simulink model "model"  (R2022a)
settings: Solver=VariableStepAuto  StartTime=0.0  StopTime=Inf  RelTol=1e-3
settings Model: Creator=mateu  LastModifiedBy=mateu

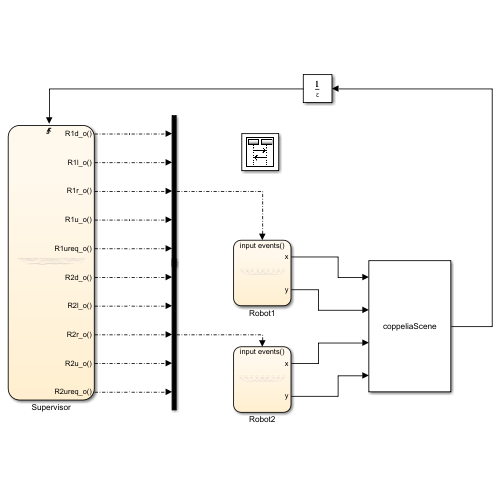
[thumbnail: Simulink's stored preview of the top-level diagram]
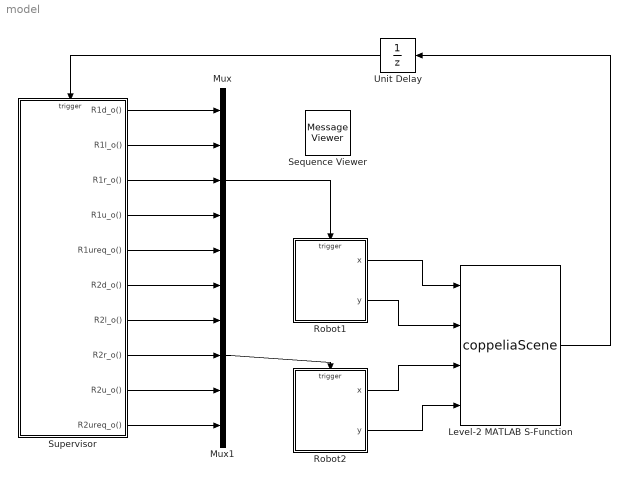
== system model ==
  Level-2 MATLAB S-Function : M-S-Function  FunctionName=coppeliaScene
  Mux : Mux  Inputs=5
  Mux1 : Mux  Inputs=5
  Robot1 : Stateflow chart  TreatAsAtomicUnit=on
  Robot2 : Stateflow chart  TreatAsAtomicUnit=on
  Sequence Viewer : MessageViewer
  Supervisor : Stateflow chart  TreatAsAtomicUnit=on
  Unit Delay : UnitDelay  SampleTime=-1  HasFrameUpgradeWarning=on
  wires:
  Level-2 MATLAB S-Function/1 -> Unit Delay/1
  Robot2/1(x) -> Level-2 MATLAB S-Function/3
  Robot2/2(y) -> Level-2 MATLAB S-Function/4
  Robot1/1(x) -> Level-2 MATLAB S-Function/1
  Robot1/2(y) -> Level-2 MATLAB S-Function/2
  Unit Delay/1 -> Supervisor/Trigger
  Mux/1 -> Robot1/Trigger
  Mux1/1 -> Robot2/Trigger
  Supervisor/1(R1d_o()) -> Mux/1
  Supervisor/2(R1l_o()) -> Mux/2
  Supervisor/3(R1r_o()) -> Mux/3
  Supervisor/4(R1u_o()) -> Mux/4
  Supervisor/5(R1ureq_o()) -> Mux/5
  Supervisor/6(R2d_o()) -> Mux1/1
  Supervisor/7(R2l_o()) -> Mux1/2
  Supervisor/8(R2r_o()) -> Mux1/3
  Supervisor/9(R2u_o()) -> Mux1/4
  Supervisor/10(R2ureq_o()) -> Mux1/5

== stateflow chart model/Robot2 ==
  settings: executeAtInitialization=1
  state s1
    x=1;
    y=1;
  state s2
    x=1;
    y=2;
  state s3
    x=1;
    y=3;
  state s4
    x=2;
    y=1;
  state s5
    x=2;
    y=2;
  state s6
    x=2;
    y=3;
  state s7
    x=3;
    y=1;
  state s8
    x=3;
    y=2;
  state s9
    x=3;
    y=3;
  (default) -> s4
  s2 -> s1 [order 1] : R2d
  s4 -> s1 [order 1] : R2l
  s1 -> s4 [order 1] : R2r
  s1 -> s2 [order 2] : R2u
  s3 -> s2 [order 1] : R2d
  s5 -> s2 [order 2] : R2l
  s2 -> s5 [order 2] : R2r
  s2 -> s3 [order 3] : R2u
  s6 -> s3 [order 2] : R2l
  s3 -> s6 [order 2] : R2r
  s5 -> s4 [order 1] : R2d
  s7 -> s4 [order 1] : R2l
  s4 -> s7 [order 2] : R2r
  s4 -> s5 [order 3] : R2u
  s6 -> s5 [order 1] : R2d
  s8 -> s5 [order 2] : R2l
  s5 -> s8 [order 3] : R2r
  s5 -> s6 [order 4] : R2u
  s5 -> s6 [order 5] : R2ureq
  s9 -> s6 [order 2] : R2l
  s6 -> s9 [order 3] : R2r
  s8 -> s7 [order 1] : R2d
  s7 -> s8 [order 2] : R2u
  s9 -> s8 [order 1] : R2d
  s8 -> s9 [order 3] : R2u
  data: x output double; y output double
  events: R2d input FUNCTION_CALL_EVENT; R2l input FUNCTION_CALL_EVENT; R2r input FUNCTION_CALL_EVENT; R2u input FUNCTION_CALL_EVENT; R2ureq input FUNCTION_CALL_EVENT

== stateflow chart model/Supervisor ==
  settings: executeAtInitialization=1
  state s1
  state s2
  state s3
  state s4
  state s5
  state s6
  state s7
  state s8
  state s9
  state s10
  state s11
  state s12
  state s13
  state s14
  state s15
  state s16
  state s17
  state s18
  state s19
  state s20
  state s21
  state s22
  state s23
  state s24
  state s25
  state s26
  state s27
  state s28
  state s29
  state s30
  state s31
  state s32
  state s33
  state s34
  state s35
  state s36
  state s37
  state s38
  state s39
  state s40
  state s41
  state s42
  state s43
  state s44
  state s45
  state s46
  state s47
  state s48
  state s49
  state s50
  state s51
  state s52
  state s53
  state s54
  state s55
  state s56
  state s57
  state s58
  state s59
  state s60
  state s61
  state s62
  state s63
  state s64
  state s65
  state s66
  state s67
  state s68
  state s69
  state s70
  (default) -> s3
  s2 -> s1 [order 2] : R2d {send(R2d_o);}
  s4 -> s1 [order 4] : R2l {send(R2l_o);}
  s25 -> s1 [order 1] : R1l {send(R1l_o);}
  s1 -> s25 [order 1] : R1r {send(R1r_o);}
  s1 -> s4 [order 2] : R2r {send(R2r_o);}
  s1 -> s2 [order 3] : R2u {send(R2u_o);}
  s5 -> s2 [order 4] : R2l {send(R2l_o);}
  s26 -> s2 [order 1] : R1l {send(R1l_o);}
  s2 -> s26 [order 1] : R1r {send(R1r_o);}
  s2 -> s5 [order 3] : R2r {send(R2r_o);}
  s4 -> s3 [order 3] : R2d {send(R2d_o);}
  s6 -> s3 [order 3] : R2l {send(R2l_o);}
  s10 -> s3 [order 1] : R1d {send(R1d_o);}
  s3 -> s10 [order 1] : R1u {send(R1u_o);}
  s3 -> s6 [order 2] : R2r {send(R2r_o);}
  s3 -> s4 [order 3] : R2u {send(R2u_o);}
  s5 -> s4 [order 3] : R2d {send(R2d_o);}
  s7 -> s4 [order 4] : R2l {send(R2l_o);}
  s11 -> s4 [order 1] : R1d {send(R1d_o);}
  s27 -> s4 [order 1] : R1l {send(R1l_o);}
  s4 -> s27 [order 1] : R1r {send(R1r_o);}
  s4 -> s11 [order 2] : R1u {send(R1u_o);}
  s4 -> s7 [order 5] : R2r {send(R2r_o);}
  s4 -> s5 [order 6] : R2u {send(R2u_o);}
  s4 -> s5 [order 7] : R2ureq {send(R2ureq_o);}
  s8 -> s5 [order 4] : R2l {send(R2l_o);}
  s12 -> s5 [order 1] : R1d {send(R1d_o);}
  s28 -> s5 [order 1] : R1l {send(R1l_o);}
  s5 -> s28 [order 1] : R1r {send(R1r_o);}
  s5 -> s12 [order 2] : R1u {send(R1u_o);}
  s5 -> s8 [order 5] : R2r {send(R2r_o);}
  s7 -> s6 [order 3] : R2d {send(R2d_o);}
  s13 -> s6 [order 1] : R1d {send(R1d_o);}
  s29 -> s6 [order 1] : R1l {send(R1l_o);}
  s6 -> s29 [order 1] : R1r {send(R1r_o);}
  s6 -> s13 [order 2] : R1u {send(R1u_o);}
  s6 -> s7 [order 4] : R2u {send(R2u_o);}
  s8 -> s7 [order 3] : R2d {send(R2d_o);}
  s14 -> s7 [order 1] : R1d {send(R1d_o);}
  s30 -> s7 [order 1] : R1l {send(R1l_o);}
  s7 -> s30 [order 1] : R1r {send(R1r_o);}
  s7 -> s14 [order 2] : R1u {send(R1u_o);}
  s7 -> s8 [order 5] : R2u {send(R2u_o);}
  s15 -> s8 [order 1] : R1d {send(R1d_o);}
  s31 -> s8 [order 1] : R1l {send(R1l_o);}
  s8 -> s31 [order 1] : R1r {send(R1r_o);}
  s8 -> s15 [order 2] : R1u {send(R1u_o);}
  s10 -> s9 [order 5] : R2l {send(R2l_o);}
  s16 -> s9 [order 1] : R1d {send(R1d_o);}
  s32 -> s9 [order 2] : R1l {send(R1l_o);}
  s9 -> s32 [order 1] : R1r {send(R1r_o);}
  s9 -> s16 [order 2] : R1u {send(R1u_o);}
  s9 -> s16 [order 3] : R1ureq {send(R1ureq_o);}
  s9 -> s10 [order 4] : R2r {send(R2r_o);}
  s11 -> s10 [order 4] : R2d {send(R2d_o);}
  s13 -> s10 [order 5] : R2l {send(R2l_o);}
  s18 -> s10 [order 1] : R1d {send(R1d_o);}
  s35 -> s10 [order 1] : R1l {send(R1l_o);}
  s10 -> s35 [order 2] : R1r {send(R1r_o);}
  s10 -> s18 [order 3] : R1u {send(R1u_o);}
  s10 -> s18 [order 4] : R1ureq {send(R1ureq_o);}
  s10 -> s13 [order 6] : R2r {send(R2r_o);}
  s10 -> s11 [order 7] : R2u {send(R2u_o);}
  s12 -> s11 [order 5] : R2d {send(R2d_o);}
  s14 -> s11 [order 6] : R2l {send(R2l_o);}
  s19 -> s11 [order 1] : R1d {send(R1d_o);}
  s11 -> s19 [order 2] : R1u {send(R1u_o);}
  s11 -> s19 [order 3] : R1ureq {send(R1ureq_o);}
  s11 -> s14 [order 5] : R2r {send(R2r_o);}
  s11 -> s12 [order 6] : R2u {send(R2u_o);}
  s11 -> s12 [order 7] : R2ureq {send(R2ureq_o);}
  s15 -> s12 [order 6] : R2l {send(R2l_o);}
  s20 -> s12 [order 1] : R1d {send(R1d_o);}
  s36 -> s12 [order 2] : R1l {send(R1l_o);}
  s12 -> s36 [order 2] : R1r {send(R1r_o);}
  s12 -> s20 [order 3] : R1u {send(R1u_o);}
  s12 -> s20 [order 4] : R1ureq {send(R1ureq_o);}
  s12 -> s15 [order 6] : R2r {send(R2r_o);}
  s14 -> s13 [order 5] : R2d {send(R2d_o);}
  s21 -> s13 [order 1] : R1d {send(R1d_o);}
  s37 -> s13 [order 2] : R1l {send(R1l_o);}
  s13 -> s37 [order 2] : R1r {send(R1r_o);}
  s13 -> s21 [order 3] : R1u {send(R1u_o);}
  s13 -> s21 [order 4] : R1ureq {send(R1ureq_o);}
  s13 -> s14 [order 6] : R2u {send(R2u_o);}
  s15 -> s14 [order 5] : R2d {send(R2d_o);}
  s22 -> s14 [order 1] : R1d {send(R1d_o);}
  s38 -> s14 [order 2] : R1l {send(R1l_o);}
  s14 -> s38 [order 2] : R1r {send(R1r_o);}
  s14 -> s22 [order 3] : R1u {send(R1u_o);}
  s14 -> s22 [order 4] : R1ureq {send(R1ureq_o);}
  s14 -> s15 [order 7] : R2u {send(R2u_o);}
  s23 -> s15 [order 1] : R1d {send(R1d_o);}
  s39 -> s15 [order 2] : R1l {send(R1l_o);}
  s15 -> s39 [order 2] : R1r {send(R1r_o);}
  s15 -> s23 [order 3] : R1u {send(R1u_o);}
  s15 -> s23 [order 4] : R1ureq {send(R1ureq_o);}
  s17 -> s16 [order 2] : R2d {send(R2d_o);}
  s18 -> s16 [order 3] : R2l {send(R2l_o);}
  s40 -> s16 [order 2] : R1l {send(R1l_o);}
  s16 -> s40 [order 2] : R1r {send(R1r_o);}
  s16 -> s18 [order 3] : R2r {send(R2r_o);}
  s16 -> s17 [order 4] : R2u {send(R2u_o);}
  s19 -> s17 [order 3] : R2l {send(R2l_o);}
  s41 -> s17 [order 2] : R1l {send(R1l_o);}
  s17 -> s41 [order 1] : R1r {send(R1r_o);}
  s17 -> s19 [order 3] : R2r {send(R2r_o);}
  s19 -> s18 [order 2] : R2d {send(R2d_o);}
  s21 -> s18 [order 3] : R2l {send(R2l_o);}
  s43 -> s18 [order 2] : R1l {send(R1l_o);}
  s18 -> s43 [order 2] : R1r {send(R1r_o);}
  s18 -> s21 [order 4] : R2r {send(R2r_o);}
  s18 -> s19 [order 5] : R2u {send(R2u_o);}
  s20 -> s19 [order 2] : R2d {send(R2d_o);}
  s22 -> s19 [order 4] : R2l {send(R2l_o);}
  s19 -> s22 [order 4] : R2r {send(R2r_o);}
  s19 -> s20 [order 5] : R2u {send(R2u_o);}
  s19 -> s20 [order 6] : R2ureq {send(R2ureq_o);}
  s23 -> s20 [order 4] : R2l {send(R2l_o);}
  s20 -> s23 [order 3] : R2r {send(R2r_o);}
  s22 -> s21 [order 3] : R2d {send(R2d_o);}
  s44 -> s21 [order 2] : R1l {send(R1l_o);}
  s21 -> s44 [order 2] : R1r {send(R1r_o);}
  s21 -> s22 [order 4] : R2u {send(R2u_o);}
  s23 -> s22 [order 3] : R2d {send(R2d_o);}
  s45 -> s22 [order 2] : R1l {send(R1l_o);}
  s22 -> s45 [order 2] : R1r {send(R1r_o);}
  s22 -> s23 [order 5] : R2u {send(R2u_o);}
  s46 -> s23 [order 2] : R1l {send(R1l_o);}
  s23 -> s46 [order 2] : R1r {send(R1r_o);}
  s25 -> s24 [order 4] : R2d {send(R2d_o);}
  s32 -> s24 [order 1] : R1d {send(R1d_o);}
  s47 -> s24 [order 1] : R1l {send(R1l_o);}
  s24 -> s47 [order 1] : R1r {send(R1r_o);}
  s24 -> s32 [order 2] : R1u {send(R1u_o);}
  s24 -> s25 [order 3] : R2u {send(R2u_o);}
  s26 -> s25 [order 4] : R2d {send(R2d_o);}
  s27 -> s25 [order 3] : R2l {send(R2l_o);}
  s33 -> s25 [order 1] : R1d {send(R1d_o);}
  s48 -> s25 [order 1] : R1l {send(R1l_o);}
  s25 -> s48 [order 2] : R1r {send(R1r_o);}
  s25 -> s33 [order 3] : R1u {send(R1u_o);}
  s25 -> s27 [order 5] : R2r {send(R2r_o);}
  s25 -> s26 [order 6] : R2u {send(R2u_o);}
  s28 -> s26 [order 5] : R2l {send(R2l_o);}
  s34 -> s26 [order 1] : R1d {send(R1d_o);}
  s49 -> s26 [order 1] : R1l {send(R1l_o);}
  s26 -> s49 [order 2] : R1r {send(R1r_o);}
  s26 -> s34 [order 3] : R1u {send(R1u_o);}
  s26 -> s28 [order 5] : R2r {send(R2r_o);}
  s28 -> s27 [order 4] : R2d {send(R2d_o);}
  s30 -> s27 [order 5] : R2l {send(R2l_o);}
  s51 -> s27 [order 1] : R1l {send(R1l_o);}
  s27 -> s51 [order 2] : R1r {send(R1r_o);}
  s27 -> s30 [order 4] : R2r {send(R2r_o);}
  s27 -> s28 [order 5] : R2u {send(R2u_o);}
  s27 -> s28 [order 6] : R2ureq {send(R2ureq_o);}
  s31 -> s28 [order 5] : R2l {send(R2l_o);}
  s36 -> s28 [order 1] : R1d {send(R1d_o);}
  s52 -> s28 [order 1] : R1l {send(R1l_o);}
  s28 -> s52 [order 2] : R1r {send(R1r_o);}
  s28 -> s36 [order 3] : R1u {send(R1u_o);}
  s28 -> s31 [order 6] : R2r {send(R2r_o);}
  s30 -> s29 [order 4] : R2d {send(R2d_o);}
  s37 -> s29 [order 1] : R1d {send(R1d_o);}
  s29 -> s37 [order 2] : R1u {send(R1u_o);}
  s29 -> s30 [order 3] : R2u {send(R2u_o);}
  s31 -> s30 [order 4] : R2d {send(R2d_o);}
  s38 -> s30 [order 1] : R1d {send(R1d_o);}
  s53 -> s30 [order 1] : R1l {send(R1l_o);}
  s30 -> s53 [order 2] : R1r {send(R1r_o);}
  s30 -> s38 [order 3] : R1u {send(R1u_o);}
  s30 -> s31 [order 6] : R2u {send(R2u_o);}
  s39 -> s31 [order 1] : R1d {send(R1d_o);}
  s54 -> s31 [order 1] : R1l {send(R1l_o);}
  s31 -> s54 [order 2] : R1r {send(R1r_o);}
  s31 -> s39 [order 3] : R1u {send(R1u_o);}
  s33 -> s32 [order 4] : R2d {send(R2d_o);}
  s35 -> s32 [order 4] : R2l {send(R2l_o);}
  s40 -> s32 [order 1] : R1d {send(R1d_o);}
  s55 -> s32 [order 2] : R1l {send(R1l_o);}
  s32 -> s55 [order 3] : R1r {send(R1r_o);}
  s32 -> s40 [order 4] : R1u {send(R1u_o);}
  s32 -> s35 [order 5] : R2r {send(R2r_o);}
  s32 -> s33 [order 6] : R2u {send(R2u_o);}
  s34 -> s33 [order 4] : R2d {send(R2d_o);}
  s41 -> s33 [order 1] : R1d {send(R1d_o);}
  s56 -> s33 [order 2] : R1l {send(R1l_o);}
  s33 -> s56 [order 2] : R1r {send(R1r_o);}
  s33 -> s41 [order 3] : R1u {send(R1u_o);}
  s33 -> s34 [order 5] : R2u {send(R2u_o);}
  s36 -> s34 [order 4] : R2l {send(R2l_o);}
  s42 -> s34 [order 1] : R1d {send(R1d_o);}
  s57 -> s34 [order 2] : R1l {send(R1l_o);}
  s34 -> s57 [order 2] : R1r {send(R1r_o);}
  s34 -> s42 [order 3] : R1u {send(R1u_o);}
  s34 -> s36 [order 5] : R2r {send(R2r_o);}
  s37 -> s35 [order 5] : R2l {send(R2l_o);}
  s43 -> s35 [order 1] : R1d {send(R1d_o);}
  s58 -> s35 [order 2] : R1l {send(R1l_o);}
  s35 -> s58 [order 2] : R1r {send(R1r_o);}
  s35 -> s43 [order 3] : R1u {send(R1u_o);}
  s35 -> s37 [order 5] : R2r {send(R2r_o);}
  s39 -> s36 [order 6] : R2l {send(R2l_o);}
  s60 -> s36 [order 2] : R1l {send(R1l_o);}
  s36 -> s60 [order 3] : R1r {send(R1r_o);}
  s36 -> s39 [order 5] : R2r {send(R2r_o);}
  s38 -> s37 [order 4] : R2d {send(R2d_o);}
  s44 -> s37 [order 1] : R1d {send(R1d_o);}
  s61 -> s37 [order 1] : R1l {send(R1l_o);}
  s37 -> s61 [order 3] : R1r {send(R1r_o);}
  s37 -> s44 [order 4] : R1u {send(R1u_o);}
  s37 -> s38 [order 6] : R2u {send(R2u_o);}
  s39 -> s38 [order 5] : R2d {send(R2d_o);}
  s45 -> s38 [order 1] : R1d {send(R1d_o);}
  s38 -> s45 [order 3] : R1u {send(R1u_o);}
  s38 -> s39 [order 5] : R2u {send(R2u_o);}
  s46 -> s39 [order 1] : R1d {send(R1d_o);}
  s62 -> s39 [order 2] : R1l {send(R1l_o);}
  s39 -> s62 [order 3] : R1r {send(R1r_o);}
  s39 -> s46 [order 4] : R1u {send(R1u_o);}
  s41 -> s40 [order 4] : R2d {send(R2d_o);}
  s43 -> s40 [order 4] : R2l {send(R2l_o);}
  s63 -> s40 [order 2] : R1l {send(R1l_o);}
  s40 -> s63 [order 3] : R1r {send(R1r_o);}
  s40 -> s43 [order 4] : R2r {send(R2r_o);}
  s40 -> s41 [order 5] : R2u {send(R2u_o);}
  s42 -> s41 [order 3] : R2d {send(R2d_o);}
  s64 -> s41 [order 2] : R1l {send(R1l_o);}
  s41 -> s64 [order 3] : R1r {send(R1r_o);}
  s41 -> s42 [order 5] : R2u {send(R2u_o);}
  s65 -> s42 [order 2] : R1l {send(R1l_o);}
  s42 -> s65 [order 2] : R1r {send(R1r_o);}
  s44 -> s43 [order 4] : R2l {send(R2l_o);}
  s66 -> s43 [order 2] : R1l {send(R1l_o);}
  s43 -> s66 [order 3] : R1r {send(R1r_o);}
  s43 -> s44 [order 5] : R2r {send(R2r_o);}
  s45 -> s44 [order 4] : R2d {send(R2d_o);}
  s69 -> s44 [order 2] : R1l {send(R1l_o);}
  s44 -> s69 [order 3] : R1r {send(R1r_o);}
  s44 -> s45 [order 5] : R2u {send(R2u_o);}
  s46 -> s45 [order 3] : R2d {send(R2d_o);}
  s70 -> s45 [order 1] : R1l {send(R1l_o);}
  s45 -> s70 [order 3] : R1r {send(R1r_o);}
  s45 -> s46 [order 5] : R2u {send(R2u_o);}
  s48 -> s47 [order 3] : R2d {send(R2d_o);}
  s50 -> s47 [order 2] : R2l {send(R2l_o);}
  s55 -> s47 [order 1] : R1d {send(R1d_o);}
  s47 -> s55 [order 2] : R1u {send(R1u_o);}
  s47 -> s50 [order 3] : R2r {send(R2r_o);}
  s47 -> s48 [order 4] : R2u {send(R2u_o);}
  s49 -> s48 [order 3] : R2d {send(R2d_o);}
  s51 -> s48 [order 4] : R2l {send(R2l_o);}
  s56 -> s48 [order 1] : R1d {send(R1d_o);}
  s48 -> s56 [order 2] : R1u {send(R1u_o);}
  s48 -> s51 [order 4] : R2r {send(R2r_o);}
  s48 -> s49 [order 5] : R2u {send(R2u_o);}
  s52 -> s49 [order 4] : R2l {send(R2l_o);}
  s57 -> s49 [order 1] : R1d {send(R1d_o);}
  s49 -> s57 [order 2] : R1u {send(R1u_o);}
  s49 -> s52 [order 4] : R2r {send(R2r_o);}
  s51 -> s50 [order 3] : R2d {send(R2d_o);}
  s58 -> s50 [order 1] : R1d {send(R1d_o);}
  s50 -> s58 [order 1] : R1u {send(R1u_o);}
  s50 -> s51 [order 3] : R2u {send(R2u_o);}
  s52 -> s51 [order 3] : R2d {send(R2d_o);}
  s53 -> s51 [order 2] : R2l {send(R2l_o);}
  s59 -> s51 [order 1] : R1d {send(R1d_o);}
  s51 -> s59 [order 2] : R1u {send(R1u_o);}
  s51 -> s53 [order 5] : R2r {send(R2r_o);}
  s51 -> s52 [order 6] : R2u {send(R2u_o);}
  s51 -> s52 [order 7] : R2ureq {send(R2ureq_o);}
  s54 -> s52 [order 4] : R2l {send(R2l_o);}
  s60 -> s52 [order 1] : R1d {send(R1d_o);}
  s52 -> s60 [order 2] : R1u {send(R1u_o);}
  s52 -> s54 [order 5] : R2r {send(R2r_o);}
  s54 -> s53 [order 3] : R2d {send(R2d_o);}
  s53 -> s54 [order 3] : R2u {send(R2u_o);}
  s62 -> s54 [order 1] : R1d {send(R1d_o);}
  s54 -> s62 [order 2] : R1u {send(R1u_o);}
  s56 -> s55 [order 4] : R2d {send(R2d_o);}
  s58 -> s55 [order 4] : R2l {send(R2l_o);}
  s63 -> s55 [order 1] : R1d {send(R1d_o);}
  s55 -> s63 [order 3] : R1u {send(R1u_o);}
  s55 -> s58 [order 4] : R2r {send(R2r_o);}
  s55 -> s56 [order 5] : R2u {send(R2u_o);}
  s57 -> s56 [order 4] : R2d {send(R2d_o);}
  s59 -> s56 [order 4] : R2l {send(R2l_o);}
  s64 -> s56 [order 1] : R1d {send(R1d_o);}
  s56 -> s64 [order 3] : R1u {send(R1u_o);}
  s56 -> s59 [order 5] : R2r {send(R2r_o);}
  s56 -> s57 [order 6] : R2u {send(R2u_o);}
  s60 -> s57 [order 5] : R2l {send(R2l_o);}
  s65 -> s57 [order 1] : R1d {send(R1d_o);}
  s57 -> s65 [order 3] : R1u {send(R1u_o);}
  s57 -> s60 [order 5] : R2r {send(R2r_o);}
  s59 -> s58 [order 3] : R2d {send(R2d_o);}
  s61 -> s58 [order 3] : R2l {send(R2l_o);}
  s66 -> s58 [order 1] : R1d {send(R1d_o);}
  s58 -> s66 [order 3] : R1u {send(R1u_o);}
  s58 -> s61 [order 5] : R2r {send(R2r_o);}
  s58 -> s59 [order 6] : R2u {send(R2u_o);}
  s60 -> s59 [order 4] : R2d {send(R2d_o);}
  s67 -> s59 [order 1] : R1d {send(R1d_o);}
  s59 -> s67 [order 2] : R1u {send(R1u_o);}
  s59 -> s60 [order 5] : R2u {send(R2u_o);}
  s59 -> s60 [order 6] : R2ureq {send(R2ureq_o);}
  s62 -> s60 [order 3] : R2l {send(R2l_o);}
  s68 -> s60 [order 1] : R1d {send(R1d_o);}
  s60 -> s68 [order 3] : R1u {send(R1u_o);}
  s60 -> s62 [order 6] : R2r {send(R2r_o);}
  s69 -> s61 [order 1] : R1d {send(R1d_o);}
  s61 -> s69 [order 2] : R1u {send(R1u_o);}
  s64 -> s63 [order 3] : R2d {send(R2d_o);}
  s66 -> s63 [order 3] : R2l {send(R2l_o);}
  s63 -> s66 [order 3] : R2r {send(R2r_o);}
  s63 -> s64 [order 4] : R2u {send(R2u_o);}
  s65 -> s64 [order 3] : R2d {send(R2d_o);}
  s67 -> s64 [order 3] : R2l {send(R2l_o);}
  s64 -> s67 [order 4] : R2r {send(R2r_o);}
  s64 -> s65 [order 5] : R2u {send(R2u_o);}
  s68 -> s65 [order 3] : R2l {send(R2l_o);}
  s65 -> s68 [order 4] : R2r {send(R2r_o);}
  s67 -> s66 [order 2] : R2d {send(R2d_o);}
  s69 -> s66 [order 3] : R2l {send(R2l_o);}
  s66 -> s69 [order 4] : R2r {send(R2r_o);}
  s66 -> s67 [order 5] : R2u {send(R2u_o);}
  s68 -> s67 [order 2] : R2d {send(R2d_o);}
  s70 -> s67 [order 3] : R2l {send(R2l_o);}
  s67 -> s70 [order 4] : R2r {send(R2r_o);}
  s67 -> s68 [order 5] : R2u {send(R2u_o);}
  s67 -> s68 [order 6] : R2ureq {send(R2ureq_o);}
  s70 -> s69 [order 2] : R2d {send(R2d_o);}
  s69 -> s70 [order 4] : R2u {send(R2u_o);}
  events: R1d input RISING_EDGE_EVENT; R1d_o output FUNCTION_CALL_EVENT; R1l input RISING_EDGE_EVENT; R1l_o output FUNCTION_CALL_EVENT; R1r input RISING_EDGE_EVENT; R1r_o output FUNCTION_CALL_EVENT; R1u input RISING_EDGE_EVENT; R1u_o output FUNCTION_CALL_EVENT; R1ureq input RISING_EDGE_EVENT; R1ureq_o output FUNCTION_CALL_EVENT; R2d input RISING_EDGE_EVENT; R2d_o output FUNCTION_CALL_EVENT; R2l input RISING_EDGE_EVENT; R2l_o output FUNCTION_CALL_EVENT; R2r input RISING_EDGE_EVENT; R2r_o output FUNCTION_CALL_EVENT; R2u input RISING_EDGE_EVENT; R2u_o output FUNCTION_CALL_EVENT; R2ureq input RISING_EDGE_EVENT; R2ureq_o output FUNCTION_CALL_EVENT

== stateflow chart model/Robot1 ==
  settings: executeAtInitialization=1
  state s1
    x=1;
    y=1;
  state s2
    x=1;
    y=2;
  state s3
    x=1;
    y=3;
  state s4
    x=2;
    y=1;
  state s5
    x=2;
    y=2;
  state s6
    x=2;
    y=3;
  state s7
    x=3;
    y=1;
  state s8
    x=3;
    y=2;
  state s9
    x=3;
    y=3;
  (default) -> s1
  s2 -> s1 [order 1] : R1d
  s4 -> s1 [order 1] : R1l
  s1 -> s4 [order 1] : R1r
  s1 -> s2 [order 2] : R1u
  s3 -> s2 [order 1] : R1d
  s5 -> s2 [order 2] : R1l
  s2 -> s5 [order 2] : R1r
  s2 -> s3 [order 3] : R1u
  s2 -> s3 [order 4] : R1ureq
  s6 -> s3 [order 2] : R1l
  s3 -> s6 [order 2] : R1r
  s5 -> s4 [order 1] : R1d
  s7 -> s4 [order 1] : R1l
  s4 -> s7 [order 2] : R1r
  s4 -> s5 [order 3] : R1u
  s6 -> s5 [order 1] : R1d
  s8 -> s5 [order 2] : R1l
  s5 -> s8 [order 3] : R1r
  s5 -> s6 [order 4] : R1u
  s9 -> s6 [order 2] : R1l
  s6 -> s9 [order 3] : R1r
  s8 -> s7 [order 1] : R1d
  s7 -> s8 [order 2] : R1u
  s9 -> s8 [order 1] : R1d
  s8 -> s9 [order 3] : R1u
  data: x output double; y output double
  events: R1d input FUNCTION_CALL_EVENT; R1l input FUNCTION_CALL_EVENT; R1r input FUNCTION_CALL_EVENT; R1u input FUNCTION_CALL_EVENT; R1ureq input FUNCTION_CALL_EVENT
